simulink model "AI_Based_Smart_HVAC_Controller"  (R2016a)
settings: Solver=FixedStepDiscrete  StartTime=0.0  StopTime=10.0  FixedStep=0.01  RelTol=1e-3
values from neighbouring files (symbols this model uses):
  AI_Enable = Simulink.Parameter    [ROM.m]
  Airflow_Defrost = Simulink.Parameter    [ROM.m]
  Airflow_Face = Simulink.Parameter    [ROM.m]
  Airflow_FaceFoot = Simulink.Parameter    [ROM.m]
  Airflow_Foot = Simulink.Parameter    [ROM.m]
  Airflow_OFF = Simulink.Parameter    [ROM.m]
  Blower_OFF_Level = Simulink.Parameter    [ROM.m]
  High_Level = Simulink.Parameter    [ROM.m]
  HVAC_Enable_OFF = Simulink.Parameter    [ROM.m]
  HVAC_Enable_ON = Simulink.Parameter    [ROM.m]
  Max_Level = Simulink.Parameter    [ROM.m]
  Medium_Level = Simulink.Parameter    [ROM.m]
libraries: simulink x2
settings Model: Creator=HP  LastModifiedBy=HP

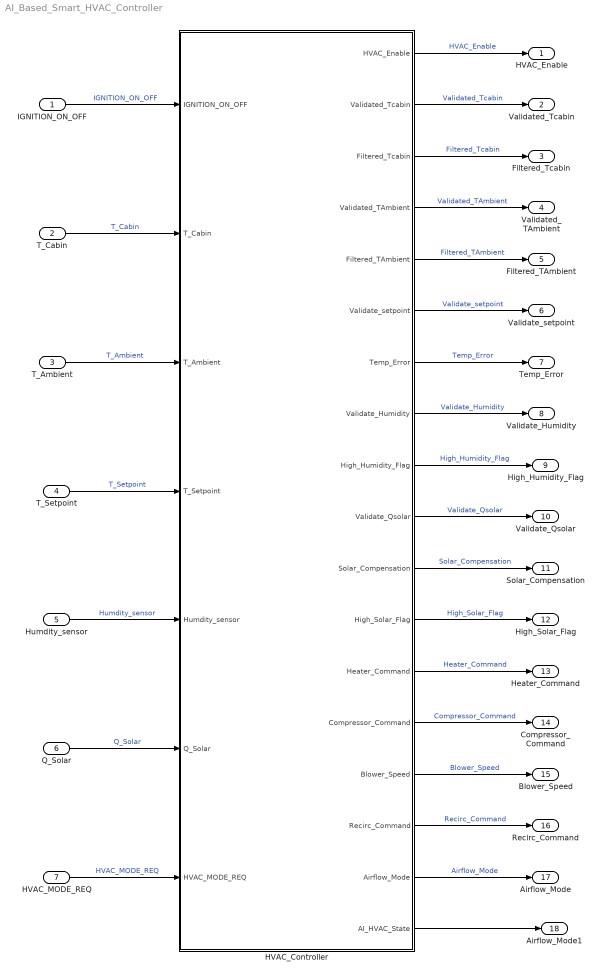
== system AI_Based_Smart_HVAC_Controller ==
  IGNITION_ON_OFF : Inport
  T_Cabin : Inport  Port=2
  T_Ambient : Inport  Port=3
  T_Setpoint : Inport  Port=4
  Humdity_sensor : Inport  Port=5
  Q_Solar : Inport  Port=6
  HVAC_MODE_REQ : Inport  Port=7
  HVAC_Controller : Subsystem
  HVAC_Enable : Outport
  Validated_Tcabin : Outport  Port=2
  Filtered_Tcabin : Outport  Port=3
  Validated_TAmbient : Outport  Port=4
  Filtered_TAmbient : Outport  Port=5
  Validate_setpoint : Outport  Port=6
  Temp_Error : Outport  Port=7
  Validate_Humidity : Outport  Port=8
  High_Humidity_Flag : Outport  Port=9
  Validate_Qsolar : Outport  Port=10
  Solar_Compensation : Outport  Port=11
  High_Solar_Flag : Outport  Port=12
  Heater_Command : Outport  Port=13
  Compressor_Command : Outport  Port=14
  Blower_Speed : Outport  Port=15
  Recirc_Command : Outport  Port=16
  Airflow_Mode : Outport  Port=17
  Airflow_Mode1 : Outport  Port=18
  wires:
  IGNITION_ON_OFF/1 -> HVAC_Controller/1(IGNITION_ON_OFF)  "IGNITION_ON_OFF"
  T_Cabin/1 -> HVAC_Controller/2(T_Cabin)  "T_Cabin"
  T_Setpoint/1 -> HVAC_Controller/4(T_Setpoint)  "T_Setpoint"
  T_Ambient/1 -> HVAC_Controller/3(T_Ambient)  "T_Ambient"
  Humdity_sensor/1 -> HVAC_Controller/5(Humdity_sensor)  "Humdity_sensor"
  Q_Solar/1 -> HVAC_Controller/6(Q_Solar)  "Q_Solar"
  HVAC_MODE_REQ/1 -> HVAC_Controller/7(HVAC_MODE_REQ)  "HVAC_MODE_REQ"
  HVAC_Controller/1(HVAC_Enable) -> HVAC_Enable/1  "HVAC_Enable"
  HVAC_Controller/2(Validated_Tcabin) -> Validated_Tcabin/1  "Validated_Tcabin"
  HVAC_Controller/3(Filtered_Tcabin) -> Filtered_Tcabin/1  "Filtered_Tcabin"
  HVAC_Controller/4(Validated_TAmbient) -> Validated_TAmbient/1  "Validated_TAmbient"
  HVAC_Controller/5(Filtered_TAmbient) -> Filtered_TAmbient/1  "Filtered_TAmbient"
  HVAC_Controller/6(Validate_setpoint) -> Validate_setpoint/1  "Validate_setpoint"
  HVAC_Controller/7(Temp_Error) -> Temp_Error/1  "Temp_Error"
  HVAC_Controller/8(Validate_Humidity) -> Validate_Humidity/1  "Validate_Humidity"
  HVAC_Controller/9(High_Humidity_Flag) -> High_Humidity_Flag/1  "High_Humidity_Flag"
  HVAC_Controller/11(Solar_Compensation) -> Solar_Compensation/1  "Solar_Compensation"
  HVAC_Controller/10(Validate_Qsolar) -> Validate_Qsolar/1  "Validate_Qsolar"
  HVAC_Controller/12(High_Solar_Flag) -> High_Solar_Flag/1  "High_Solar_Flag"
  HVAC_Controller/13(Heater_Command) -> Heater_Command/1  "Heater_Command"
  HVAC_Controller/14(Compressor_Command) -> Compressor_Command/1  "Compressor_Command"
  HVAC_Controller/15(Blower_Speed) -> Blower_Speed/1  "Blower_Speed"
  HVAC_Controller/16(Recirc_Command) -> Recirc_Command/1  "Recirc_Command"
  HVAC_Controller/17(Airflow_Mode) -> Airflow_Mode/1  "Airflow_Mode"
  HVAC_Controller/18(AI_HVAC_State) -> Airflow_Mode1/1

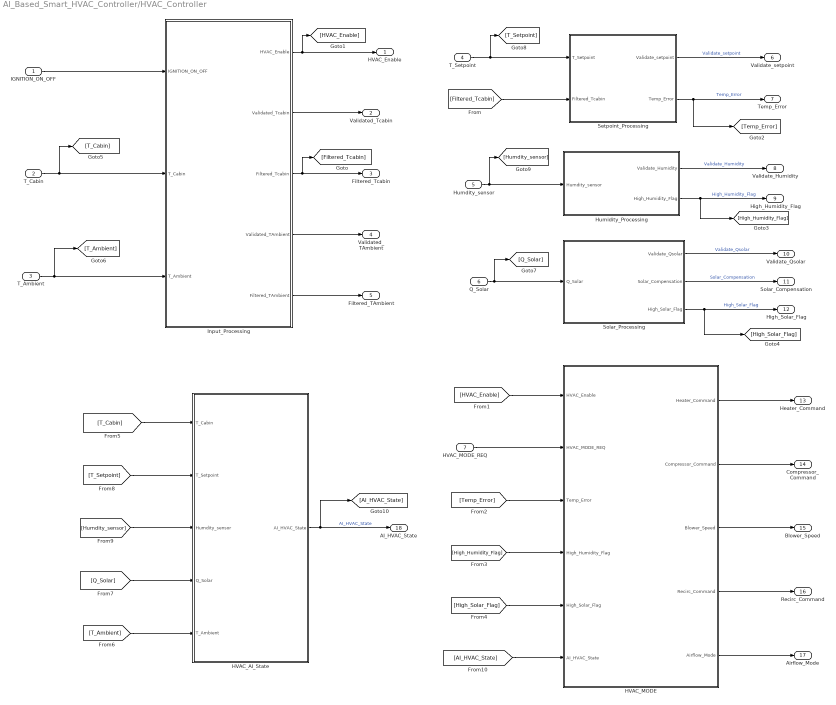
== system AI_Based_Smart_HVAC_Controller/HVAC_Controller ==
  IGNITION_ON_OFF : Inport
  T_Cabin : Inport  Port=2
  T_Ambient : Inport  Port=3
  T_Setpoint : Inport  Port=4
  Humdity_sensor : Inport  Port=5
  Q_Solar : Inport  Port=6
  HVAC_MODE_REQ : Inport  Port=7
  HVAC_AI_State : Subsystem
  HVAC_MODE : Subsystem
  Humidity_Processing : Subsystem
  Input_Processing : Subsystem
  Setpoint_Processing : Subsystem
  Solar_Processing : Subsystem
  HVAC_Enable : Outport
  Validated_Tcabin : Outport  Port=2
  Filtered_Tcabin : Outport  Port=3
  Validated_TAmbient : Outport  Port=4
  Filtered_TAmbient : Outport  Port=5
  Validate_setpoint : Outport  Port=6
  Temp_Error : Outport  Port=7
  Validate_Humidity : Outport  Port=8
  High_Humidity_Flag : Outport  Port=9
  Validate_Qsolar : Outport  Port=10
  Solar_Compensation : Outport  Port=11
  High_Solar_Flag : Outport  Port=12
  Heater_Command : Outport  Port=13
  Compressor_Command : Outport  Port=14
  Blower_Speed : Outport  Port=15
  Recirc_Command : Outport  Port=16
  Airflow_Mode : Outport  Port=17
  AI_HVAC_State : Outport  Port=18
  wires:
  [High_Solar_Flag] -> HVAC_MODE/5(High_Solar_Flag)
  [HVAC_Enable] -> HVAC_MODE/1(HVAC_Enable)
  HVAC_MODE_REQ/1 -> HVAC_MODE/2(HVAC_MODE_REQ)
  [High_Humidity_Flag] -> HVAC_MODE/4(High_Humidity_Flag)
  HVAC_MODE/4(Recirc_Command) -> Recirc_Command/1
  HVAC_MODE/5(Airflow_Mode) -> Airflow_Mode/1
  HVAC_MODE/3(Blower_Speed) -> Blower_Speed/1
  HVAC_MODE/2(Compressor_Command) -> Compressor_Command/1
  [Temp_Error] -> HVAC_MODE/3(Temp_Error)
  Input_Processing/2(Validated_Tcabin) -> Validated_Tcabin/1
  Input_Processing/3(Filtered_Tcabin) -> Filtered_Tcabin/1, [Filtered_Tcabin]
  T_Setpoint/1 -> [T_Setpoint], Setpoint_Processing/1(T_Setpoint)
  Humidity_Processing/1(Validate_Humidity) -> Validate_Humidity/1  "Validate_Humidity"
  Setpoint_Processing/2(Temp_Error) -> Temp_Error/1, [Temp_Error]  "Temp_Error"
  [Filtered_Tcabin] -> Setpoint_Processing/2(Filtered_Tcabin)
  T_Cabin/1 -> [T_Cabin], Input_Processing/2(T_Cabin)
  T_Ambient/1 -> [T_Ambient], Input_Processing/3(T_Ambient)
  IGNITION_ON_OFF/1 -> Input_Processing/1(IGNITION_ON_OFF)
  Input_Processing/1(HVAC_Enable) -> HVAC_Enable/1, [HVAC_Enable]
  Input_Processing/5(Filtered_TAmbient) -> Filtered_TAmbient/1
  Input_Processing/4(Validated_TAmbient) -> Validated_TAmbient/1
  Setpoint_Processing/1(Validate_setpoint) -> Validate_setpoint/1  "Validate_setpoint"
  Solar_Processing/1(Validate_Qsolar) -> Validate_Qsolar/1  "Validate_Qsolar"
  Solar_Processing/2(Solar_Compensation) -> Solar_Compensation/1  "Solar_Compensation"
  Humidity_Processing/2(High_Humidity_Flag) -> High_Humidity_Flag/1, [High_Humidity_Flag]  "High_Humidity_Flag"
  Q_Solar/1 -> [Q_Solar], Solar_Processing/1(Q_Solar)
  Solar_Processing/3(High_Solar_Flag) -> High_Solar_Flag/1, [High_Solar_Flag]  "High_Solar_Flag"
  HVAC_MODE/1(Heater_Command) -> Heater_Command/1
  Humdity_sensor/1 -> [Humdity_sensor], Humidity_Processing/1(Humdity_sensor)
  [T_Cabin] -> HVAC_AI_State/1(T_Cabin)
  [T_Setpoint] -> HVAC_AI_State/2(T_Setpoint)
  [Humdity_sensor] -> HVAC_AI_State/3(Humdity_sensor)
  [Q_Solar] -> HVAC_AI_State/4(Q_Solar)
  [T_Ambient] -> HVAC_AI_State/5(T_Ambient)
  HVAC_AI_State/1(AI_HVAC_State) -> [AI_HVAC_State], AI_HVAC_State/1  "AI_HVAC_State"
  [AI_HVAC_State] -> HVAC_MODE/6(AI_HVAC_State)

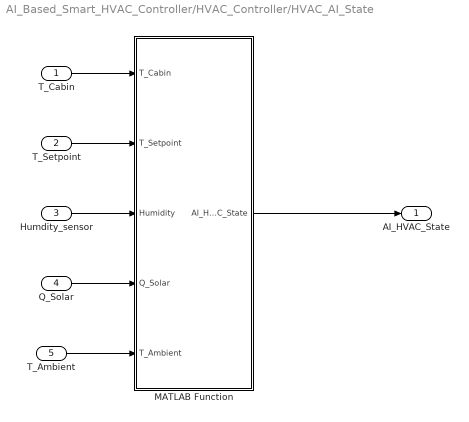
== system AI_Based_Smart_HVAC_Controller/HVAC_Controller/HVAC_AI_State ==
  T_Cabin : Inport
  T_Setpoint : Inport  Port=2
  Humdity_sensor : Inport  Port=3
  Q_Solar : Inport  Port=4
  T_Ambient : Inport  Port=5
  MATLAB Function : MATLAB Function  TreatAsAtomicUnit=on
  AI_HVAC_State : Outport
  wires:
  T_Ambient/1 -> MATLAB Function/5(T_Ambient)
  T_Setpoint/1 -> MATLAB Function/2(T_Setpoint)
  T_Cabin/1 -> MATLAB Function/1(T_Cabin)
  Humdity_sensor/1 -> MATLAB Function/3(Humidity)
  MATLAB Function/1(AI_HVAC_State) -> AI_HVAC_State/1
  Q_Solar/1 -> MATLAB Function/4(Q_Solar)

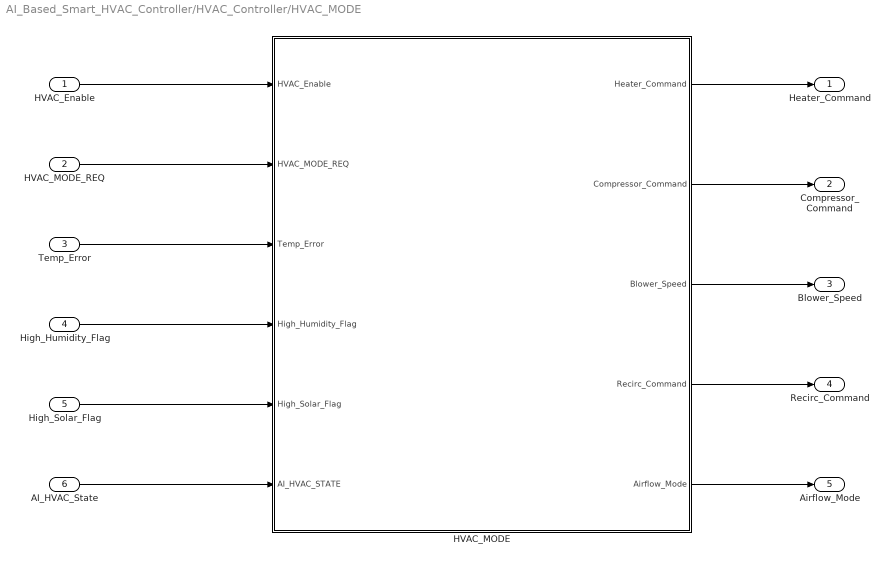
== system AI_Based_Smart_HVAC_Controller/HVAC_Controller/HVAC_MODE ==
  HVAC_Enable : Inport
  HVAC_MODE_REQ : Inport  Port=2
  Temp_Error : Inport  Port=3
  High_Humidity_Flag : Inport  Port=4
  High_Solar_Flag : Inport  Port=5
  AI_HVAC_State : Inport  Port=6
  HVAC_MODE : Stateflow chart  TreatAsAtomicUnit=on
  Heater_Command : Outport
  Compressor_Command : Outport  Port=2
  Blower_Speed : Outport  Port=3
  Recirc_Command : Outport  Port=4
  Airflow_Mode : Outport  Port=5
  wires:
  HVAC_MODE/5(Airflow_Mode) -> Airflow_Mode/1
  HVAC_MODE/4(Recirc_Command) -> Recirc_Command/1
  HVAC_MODE/3(Blower_Speed) -> Blower_Speed/1
  HVAC_MODE/2(Compressor_Command) -> Compressor_Command/1
  HVAC_MODE/1(Heater_Command) -> Heater_Command/1
  HVAC_Enable/1 -> HVAC_MODE/1(HVAC_Enable)
  HVAC_MODE_REQ/1 -> HVAC_MODE/2(HVAC_MODE_REQ)
  Temp_Error/1 -> HVAC_MODE/3(Temp_Error)
  High_Humidity_Flag/1 -> HVAC_MODE/4(High_Humidity_Flag)
  High_Solar_Flag/1 -> HVAC_MODE/5(High_Solar_Flag)
  AI_HVAC_State/1 -> HVAC_MODE/6(AI_HVAC_STATE)

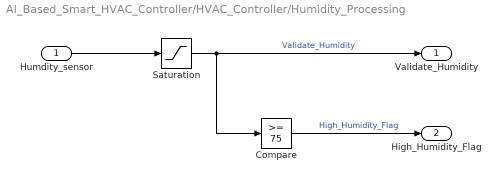
== system AI_Based_Smart_HVAC_Controller/HVAC_Controller/Humidity_Processing ==
  Humdity_sensor : Inport
  Compare : simulink/Logic and Bit Operations/Compare To Constant  relop=>=  const=75  OutDataTypeStr=boolean
  Saturation : Saturate  UpperLimit=90  LowerLimit=20
  Validate_Humidity : Outport
  High_Humidity_Flag : Outport  Port=2
  wires:
  Humdity_sensor/1 -> Saturation/1
  Compare/1 -> High_Humidity_Flag/1  "High_Humidity_Flag"
  Saturation/1 -> Validate_Humidity/1, Compare/1  "Validate_Humidity"

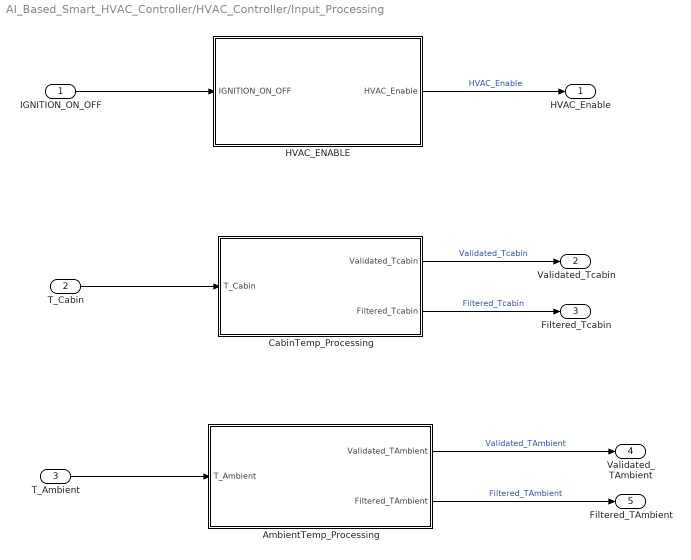
== system AI_Based_Smart_HVAC_Controller/HVAC_Controller/Input_Processing ==
  IGNITION_ON_OFF : Inport
  T_Cabin : Inport  Port=2
  T_Ambient : Inport  Port=3
  AmbientTemp_Processing : Subsystem
  CabinTemp_Processing : Subsystem
  HVAC_ENABLE : Subsystem
  HVAC_Enable : Outport
  Validated_Tcabin : Outport  Port=2
  Filtered_Tcabin : Outport  Port=3
  Validated_TAmbient : Outport  Port=4
  Filtered_TAmbient : Outport  Port=5
  wires:
  CabinTemp_Processing/2(Filtered_Tcabin) -> Filtered_Tcabin/1  "Filtered_Tcabin"
  T_Cabin/1 -> CabinTemp_Processing/1(T_Cabin)
  CabinTemp_Processing/1(Validated_Tcabin) -> Validated_Tcabin/1  "Validated_Tcabin"
  T_Ambient/1 -> AmbientTemp_Processing/1(T_Ambient)
  AmbientTemp_Processing/1(Validated_TAmbient) -> Validated_TAmbient/1  "Validated_TAmbient"
  AmbientTemp_Processing/2(Filtered_TAmbient) -> Filtered_TAmbient/1  "Filtered_TAmbient"
  IGNITION_ON_OFF/1 -> HVAC_ENABLE/1(IGNITION_ON_OFF)
  HVAC_ENABLE/1(HVAC_Enable) -> HVAC_Enable/1  "HVAC_Enable"

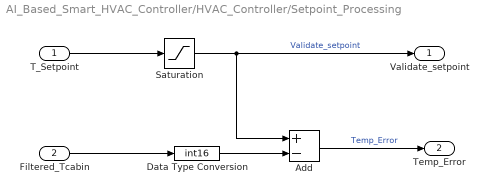
== system AI_Based_Smart_HVAC_Controller/HVAC_Controller/Setpoint_Processing ==
  T_Setpoint : Inport
  Filtered_Tcabin : Inport  Port=2
  Add : Sum  Inputs=+-
  Data Type Conversion : DataTypeConversion  OutDataTypeStr=int16
  Saturation : Saturate  UpperLimit=30  LowerLimit=18
  Validate_setpoint : Outport
  Temp_Error : Outport  Port=2
  wires:
  Filtered_Tcabin/1 -> Data Type Conversion/1
  Add/1 -> Temp_Error/1  "Temp_Error"
  Saturation/1 -> Validate_setpoint/1, Add/1  "Validate_setpoint"
  T_Setpoint/1 -> Saturation/1
  Data Type Conversion/1 -> Add/2

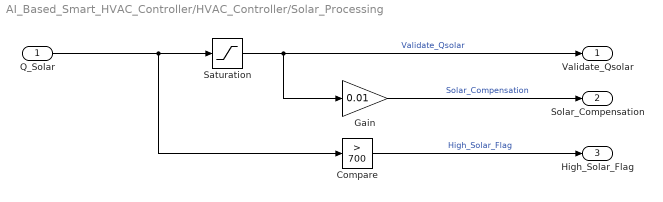
== system AI_Based_Smart_HVAC_Controller/HVAC_Controller/Solar_Processing ==
  Q_Solar : Inport
  Compare : simulink/Logic and Bit Operations/Compare To Constant  relop=>  const=700  OutDataTypeStr=boolean
  Gain : Gain  Gain=0.01
  Saturation : Saturate  UpperLimit=1000  LowerLimit=0
  Validate_Qsolar : Outport
  Solar_Compensation : Outport  Port=2
  High_Solar_Flag : Outport  Port=3
  wires:
  Q_Solar/1 -> Compare/1, Saturation/1
  Saturation/1 -> Validate_Qsolar/1, Gain/1  "Validate_Qsolar"
  Gain/1 -> Solar_Compensation/1  "Solar_Compensation"
  Compare/1 -> High_Solar_Flag/1  "High_Solar_Flag"

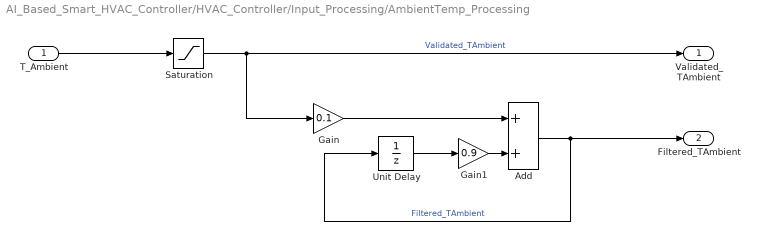
== system AI_Based_Smart_HVAC_Controller/HVAC_Controller/Input_Processing/AmbientTemp_Processing ==
  T_Ambient : Inport
  Add : Sum
  Gain : Gain  Gain=0.1
  Gain1 : Gain  Gain=0.9
  Saturation : Saturate  UpperLimit=50  LowerLimit=-10
  Unit Delay : UnitDelay  InitialCondition=30  SampleTime=-1
  Validated_TAmbient : Outport
  Filtered_TAmbient : Outport  Port=2
  wires:
  T_Ambient/1 -> Saturation/1
  Gain/1 -> Add/1
  Gain1/1 -> Add/2
  Unit Delay/1 -> Gain1/1
  Saturation/1 -> Validated_TAmbient/1, Gain/1  "Validated_TAmbient"
  Add/1 -> Filtered_TAmbient/1, Unit Delay/1  "Filtered_TAmbient"

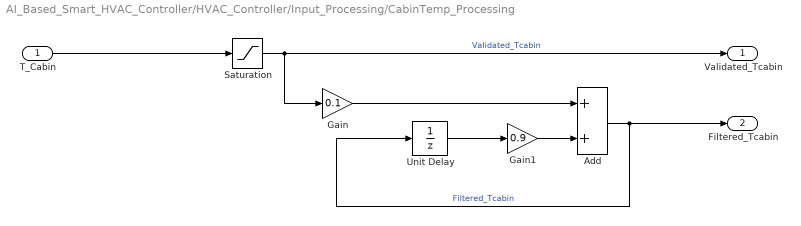
== system AI_Based_Smart_HVAC_Controller/HVAC_Controller/Input_Processing/CabinTemp_Processing ==
  T_Cabin : Inport
  Add : Sum
  Gain : Gain  Gain=0.1  RndMeth=Zero  OutDataTypeStr=Inherit: Same as input
  Gain1 : Gain  Gain=0.9  RndMeth=Zero  OutDataTypeStr=Inherit: Same as input
  Saturation : Saturate  UpperLimit=45  LowerLimit=15
  Unit Delay : UnitDelay  InitialCondition=25  SampleTime=-1
  Validated_Tcabin : Outport
  Filtered_Tcabin : Outport  Port=2
  wires:
  Saturation/1 -> Gain/1, Validated_Tcabin/1  "Validated_Tcabin"
  Unit Delay/1 -> Gain1/1
  Gain1/1 -> Add/2
  Gain/1 -> Add/1
  T_Cabin/1 -> Saturation/1
  Add/1 -> Unit Delay/1, Filtered_Tcabin/1  "Filtered_Tcabin"

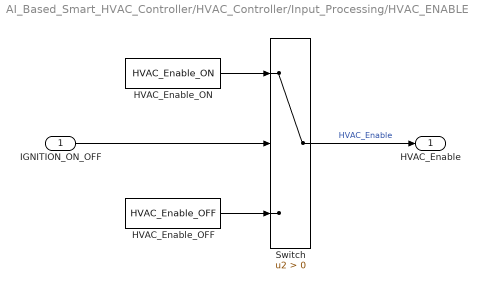
== system AI_Based_Smart_HVAC_Controller/HVAC_Controller/Input_Processing/HVAC_ENABLE ==
  IGNITION_ON_OFF : Inport
  HVAC_Enable_OFF : Constant  Value=HVAC_Enable_OFF
  HVAC_Enable_ON : Constant  Value=HVAC_Enable_ON
  Switch : Switch  Criteria=u2 > Threshold
  HVAC_Enable : Outport
  wires:
  HVAC_Enable_ON/1 -> Switch/1
  Switch/1 -> HVAC_Enable/1  "HVAC_Enable"
  HVAC_Enable_OFF/1 -> Switch/3
  IGNITION_ON_OFF/1 -> Switch/2

== matlab function AI_Based_Smart_HVAC_Controller/HVAC_Controller/HVAC_AI_State/MATLAB Function ==
  data: T_Cabin input; AI_HVAC_State output; T_Setpoint input; Humidity input; Q_Solar input; T_Ambient input
function AI_HVAC_State = AI_Controller(...
    T_Cabin,...
    T_Setpoint,...
    Humidity,...
    Q_Solar,...
    T_Ambient)

if T_Cabin > T_Setpoint + 5
    AI_HVAC_State = 3;

elseif T_Cabin > T_Setpoint + 2
    AI_HVAC_State = 2;

elseif T_Cabin < T_Setpoint - 2
    AI_HVAC_State = 4;

elseif Humidity > 80
    AI_HVAC_State = 5;

else
    AI_HVAC_State = 1;
end

== stateflow chart AI_Based_Smart_HVAC_Controller/HVAC_Controller/HVAC_MODE/HVAC_MODE ==
  state HVAC_MODE
    state HEATING
      entry:
      Heater_Command=true;
      Compressor_Command=false;
      Blower_Speed=Medium_Level;
      Recirc_Command=false;
      Airflow_Mode=Airflow_Foot;
    state IDLE
      en:
      Heater_Command=false;
      Compressor_Command=false;
      Blower_Speed=Blower_OFF_Level;
      Recirc_Command=true;
      Airflow_Mode=Airflow_FaceFoot;
    state OFF_State
      en:
      Heater_Command=false;
      Compressor_Command=false;
      Blower_Speed=Blower_OFF_Level;
      Recirc_Command=false;
      Airflow_Mode=Airflow_OFF;
    state DEFOG
      en:
      Heater_Command=true;
      Compressor_Command=true;
      Blower_Speed=High_Level;
      Recirc_Command=false;
      Airflow_Mode=Airflow_Defrost;
    state COOLING
      entry: Heater_Command=false;
      Compressor_Command=true;
      Blower_Speed=Medium_Level;
      Recirc_Command=true;
      Airflow_Mode=Airflow_Face;
    state HIGH_COOLING
      entry:
      Heater_Command=false;
      Compressor_Command=true;
      Blower_Speed=Max_Level;
      Recirc_Command=true;
      Airflow_Mode=Airflow_Face;
    (default) -> OFF_State [order 1]
    (default) -> HEATING [order 2] : [ AI_Enable==0 && Temp_Error>2 && HVAC_MODE_REQ == 2]
    IDLE -> HEATING [order 4] : [AI_Enable==1 && AI_HVAC_STATE==4]
    HEATING -> IDLE [order 2] : [Temp_Error>=-1]
    OFF_State -> IDLE : [HVAC_Enable==1 && HVAC_MODE_REQ~=0]
    HEATING -> DEFOG [order 1] : [High_Humidity_Flag ==1]
    IDLE -> OFF_State [order 1] : [HVAC_Enable==0 || HVAC_MODE_REQ==0]
    IDLE -> DEFOG [order 2] : [AI_Enable==0 && High_Humidity_Flag ==1 && Temp_Error<-2]
    IDLE -> DEFOG [order 3] : [AI_Enable==1 && AI_HVAC_STATE==5]
    DEFOG -> IDLE : [High_Humidity_Flag ==0]
    IDLE -> COOLING [order 5] : [AI_Enable==0 && Temp_Error<-2 && HVAC_MODE_REQ == 3]
    IDLE -> COOLING [order 6] : [AI_Enable==1 && (AI_HVAC_STATE==2 ||  AI_HVAC_STATE==3)]
    COOLING -> IDLE [order 2] : [Temp_Error>=- 1]
    COOLING -> DEFOG [order 1] : [High_Humidity_Flag ==1]
    HIGH_COOLING -> DEFOG [order 1] : [High_Humidity_Flag ==1]
    HIGH_COOLING -> COOLING [order 2] : [Temp_Error<-4 && High_Solar_Flag==0 ]
    COOLING -> HIGH_COOLING [order 3] : [Temp_Error<-5 || High_Solar_Flag==1 ]
  data: HVAC_Enable input; HVAC_MODE_REQ input; Temp_Error input; High_Humidity_Flag input; Heater_Command output boolean; High_Solar_Flag input; Compressor_Command output; Blower_Speed output; Recirc_Command output; Airflow_Mode output; Airflow_OFF parameter; Blower_OFF_Level parameter; Airflow_FaceFoot parameter; Medium_Level parameter; Airflow_Foot parameter; Max_Level parameter; High_Level parameter; Airflow_Defrost parameter; Airflow_Face parameter; AI_HVAC_STATE input; AI_Enable parameter
